simulink model "EngLim"  (R2018a)
settings: configuration reference "cs_ert" (kept outside this file)
settings Model: DataDictionary=EngLim.sldd  Creator=zhoutinglin  LastModifiedBy=zhoutinglin

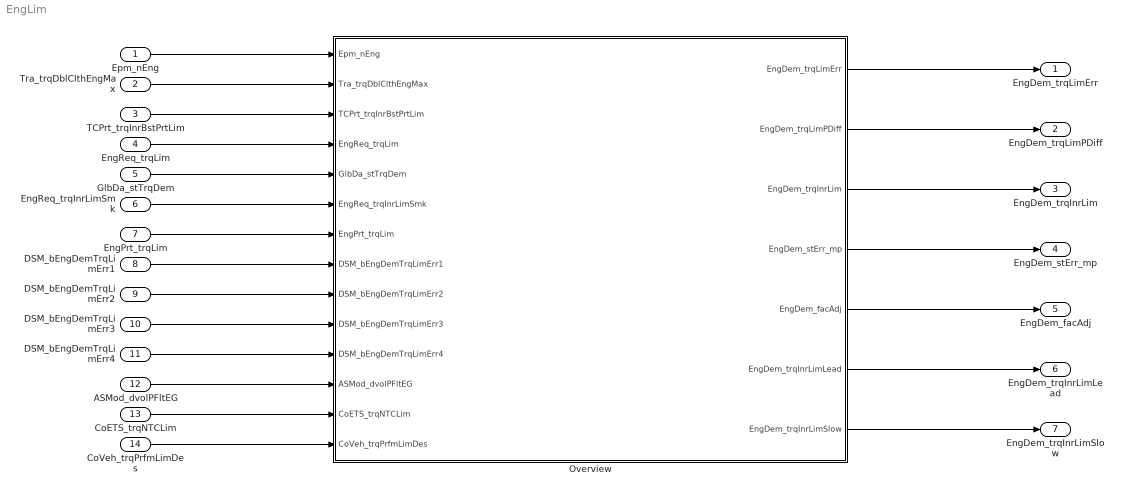
== system EngLim ==
  Epm_nEng : Inport
  Tra_trqDblClthEngMax : Inport  Port=2
  TCPrt_trqInrBstPrtLim : Inport  Port=3
  EngReq_trqLim : Inport  Port=4
  GlbDa_stTrqDem : Inport  Port=5
  EngReq_trqInrLimSmk : Inport  Port=6
  EngPrt_trqLim : Inport  Port=7
  DSM_bEngDemTrqLimErr1 : Inport  Port=8
  DSM_bEngDemTrqLimErr2 : Inport  Port=9
  DSM_bEngDemTrqLimErr3 : Inport  Port=10
  DSM_bEngDemTrqLimErr4 : Inport  Port=11
  ASMod_dvolPFltEG : Inport  Port=12
  CoETS_trqNTCLim : Inport  Port=13
  CoVeh_trqPrfmLimDes : Inport  Port=14
  Overview : Subsystem
  EngDem_trqLimErr : Outport
  EngDem_trqLimPDiff : Outport  Port=2
  EngDem_trqInrLim : Outport  Port=3
  EngDem_stErr_mp : Outport  Port=4
  EngDem_facAdj : Outport  Port=5
  EngDem_trqInrLimLead : Outport  Port=6
  EngDem_trqInrLimSlow : Outport  Port=7
  wires:
  Epm_nEng/1 -> Overview/1(Epm_nEng)
  Tra_trqDblClthEngMax/1 -> Overview/2(Tra_trqDblClthEngMax)
  TCPrt_trqInrBstPrtLim/1 -> Overview/3(TCPrt_trqInrBstPrtLim)
  EngReq_trqLim/1 -> Overview/4(EngReq_trqLim)
  GlbDa_stTrqDem/1 -> Overview/5(GlbDa_stTrqDem)
  EngReq_trqInrLimSmk/1 -> Overview/6(EngReq_trqInrLimSmk)
  EngPrt_trqLim/1 -> Overview/7(EngPrt_trqLim)
  DSM_bEngDemTrqLimErr1/1 -> Overview/8(DSM_bEngDemTrqLimErr1)
  DSM_bEngDemTrqLimErr2/1 -> Overview/9(DSM_bEngDemTrqLimErr2)
  DSM_bEngDemTrqLimErr3/1 -> Overview/10(DSM_bEngDemTrqLimErr3)
  DSM_bEngDemTrqLimErr4/1 -> Overview/11(DSM_bEngDemTrqLimErr4)
  ASMod_dvolPFltEG/1 -> Overview/12(ASMod_dvolPFltEG)
  CoETS_trqNTCLim/1 -> Overview/13(CoETS_trqNTCLim)
  CoVeh_trqPrfmLimDes/1 -> Overview/14(CoVeh_trqPrfmLimDes)
  Overview/1(EngDem_trqLimErr) -> EngDem_trqLimErr/1
  Overview/2(EngDem_trqLimPDiff) -> EngDem_trqLimPDiff/1
  Overview/3(EngDem_trqInrLim) -> EngDem_trqInrLim/1
  Overview/4(EngDem_stErr_mp) -> EngDem_stErr_mp/1
  Overview/5(EngDem_facAdj) -> EngDem_facAdj/1
  Overview/6(EngDem_trqInrLimLead) -> EngDem_trqInrLimLead/1
  Overview/7(EngDem_trqInrLimSlow) -> EngDem_trqInrLimSlow/1

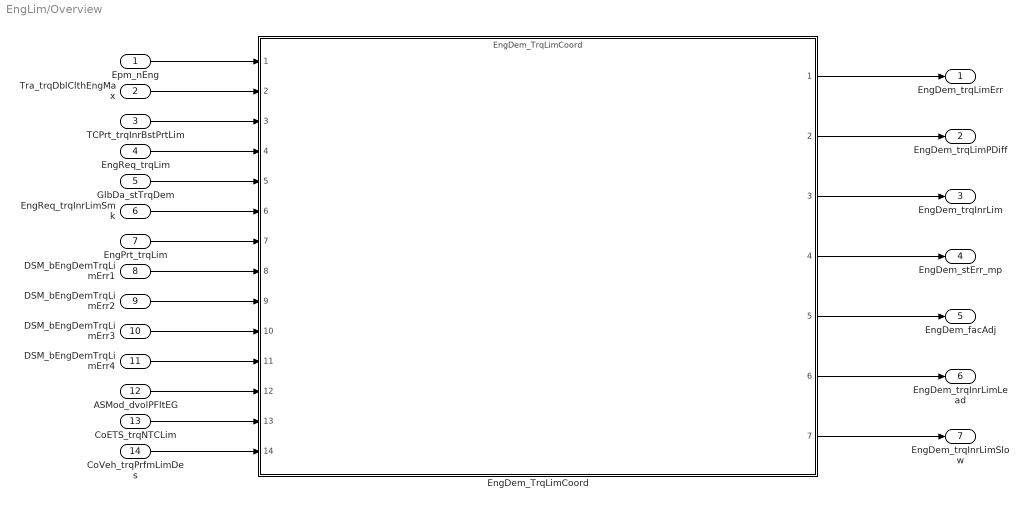
== system EngLim/Overview ==
  Epm_nEng : Inport
  Tra_trqDblClthEngMax : Inport  Port=2
  TCPrt_trqInrBstPrtLim : Inport  Port=3
  EngReq_trqLim : Inport  Port=4
  GlbDa_stTrqDem : Inport  Port=5
  EngReq_trqInrLimSmk : Inport  Port=6
  EngPrt_trqLim : Inport  Port=7
  DSM_bEngDemTrqLimErr1 : Inport  Port=8
  DSM_bEngDemTrqLimErr2 : Inport  Port=9
  DSM_bEngDemTrqLimErr3 : Inport  Port=10
  DSM_bEngDemTrqLimErr4 : Inport  Port=11
  ASMod_dvolPFltEG : Inport  Port=12
  CoETS_trqNTCLim : Inport  Port=13
  CoVeh_trqPrfmLimDes : Inport  Port=14
  EngDem_TrqLimCoord : ModelReference  ModelNameDialog=EngDem_TrqLimCoord  SimulationMode=Normal  ModelReferenceVersion=1.53
  EngDem_trqLimErr : Outport
  EngDem_trqLimPDiff : Outport  Port=2
  EngDem_trqInrLim : Outport  Port=3
  EngDem_stErr_mp : Outport  Port=4
  EngDem_facAdj : Outport  Port=5
  EngDem_trqInrLimLead : Outport  Port=6
  EngDem_trqInrLimSlow : Outport  Port=7
  wires:
  Epm_nEng/1 -> EngDem_TrqLimCoord/1
  Tra_trqDblClthEngMax/1 -> EngDem_TrqLimCoord/2
  TCPrt_trqInrBstPrtLim/1 -> EngDem_TrqLimCoord/3
  EngReq_trqLim/1 -> EngDem_TrqLimCoord/4
  GlbDa_stTrqDem/1 -> EngDem_TrqLimCoord/5
  EngReq_trqInrLimSmk/1 -> EngDem_TrqLimCoord/6
  EngPrt_trqLim/1 -> EngDem_TrqLimCoord/7
  DSM_bEngDemTrqLimErr1/1 -> EngDem_TrqLimCoord/8
  DSM_bEngDemTrqLimErr2/1 -> EngDem_TrqLimCoord/9
  DSM_bEngDemTrqLimErr3/1 -> EngDem_TrqLimCoord/10
  DSM_bEngDemTrqLimErr4/1 -> EngDem_TrqLimCoord/11
  ASMod_dvolPFltEG/1 -> EngDem_TrqLimCoord/12
  CoETS_trqNTCLim/1 -> EngDem_TrqLimCoord/13
  CoVeh_trqPrfmLimDes/1 -> EngDem_TrqLimCoord/14
  EngDem_TrqLimCoord/1 -> EngDem_trqLimErr/1
  EngDem_TrqLimCoord/2 -> EngDem_trqLimPDiff/1
  EngDem_TrqLimCoord/3 -> EngDem_trqInrLim/1
  EngDem_TrqLimCoord/4 -> EngDem_stErr_mp/1
  EngDem_TrqLimCoord/5 -> EngDem_facAdj/1
  EngDem_TrqLimCoord/6 -> EngDem_trqInrLimLead/1
  EngDem_TrqLimCoord/7 -> EngDem_trqInrLimSlow/1
